simulink model "Q2_non_idealities_added"  (R2018a)
settings: Solver=FixedStepAuto  StartTime=0.0  StopTime=2  RelTol=1e-3
libraries: powerlib x14, powerlib_meascontrol x4, pePowerMeasurement x2
settings Model: Creator=ROG  LastModifiedBy=Pc

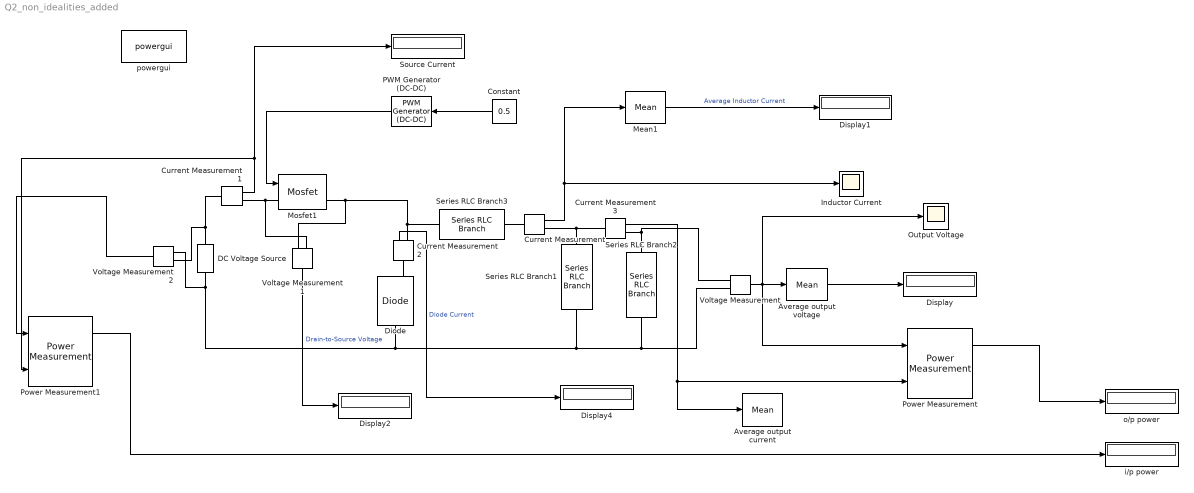
== system Q2_non_idealities_added ==
  "Average output current " : powerlib_meascontrol/Measurements/Mean  Freq=50  Vinit=0  Ts=0
  Average output voltage : powerlib_meascontrol/Measurements/Mean  Freq=50  Vinit=0  Ts=0
  Constant : Constant  Value=0.5
  Current Measurement{,1..3} (4 alike) : powerlib/Measurements/Current Measurement  PhasorSimulation=off  OutputType=Complex  PSBequivalent=0
  DC Voltage Source : powerlib/Electrical Sources/DC Voltage Source  Amplitude=56  Measurements=None
  Diode : powerlib/Power Electronics/Diode  Ron=0.001  Lon=0  Vf=0.8  IC=0  UseSnubber=0  Rs=500  Cs=250e-9  Measurements=on
  Display{,1..2,4} (4 alike) : Display
  Inductor Current : Scope
  Mean1 : powerlib_meascontrol/Measurements/Mean  Freq=50  Vinit=0  Ts=0
  Mosfet1 : powerlib/Power Electronics/Mosfet  Ron=0.022  Lon=0  Rd=0.01  Vfd=0.9  IC=0  Rs=1e5  Cs=inf  Measurements=on
  Output Voltage : Scope
  PWM Generator (DC-DC) : powerlib_meascontrol/Pulse & Signal Generators/PWM Generator (DC-DC)  Fsw=20000  Ts=0
  Power Measurement : pePowerMeasurement/Power Measurement  OverrideUsingVariant=Continuous  F=60  K=[0 1 2 3]  Ts=0
  Power Measurement1 : pePowerMeasurement/Power Measurement  OverrideUsingVariant=Continuous  F=60  K=[0 1 2 3]  Ts=0
  Series RLC Branch1 : powerlib/Elements/Series RLC Branch  LConnTagsString=__new0  RConnTagsString=__new0  BranchType=RC  Resistance=0.06  Inductance=1e-3  SetiL0=off  InitialCurrent=0  Capacitance=68e-5  Setx0=off  InitialVoltage=0  Measurements=None
  Series RLC Branch2 : powerlib/Elements/Series RLC Branch  LConnTagsString=__new0  RConnTagsString=__new0  BranchType=R  Resistance=4  Inductance=1e-3  SetiL0=off  InitialCurrent=0  Capacitance=1e-6  Setx0=off  InitialVoltage=0  Measurements=None
  Series RLC Branch3 : powerlib/Elements/Series RLC Branch  LConnTagsString=__new0  RConnTagsString=__new0  BranchType=RL  Resistance=0.064  Inductance=47e-05  SetiL0=off  InitialCurrent=0  Capacitance=1e-6  Setx0=off  InitialVoltage=0  Measurements=None
  Source Current : Display
  Voltage Measurement : powerlib/Measurements/Voltage Measurement  PhasorSimulation=off  OutputType=Complex  PSBequivalent=0
  Voltage Measurement1 : powerlib/Measurements/Voltage Measurement  PhasorSimulation=off  OutputType=Complex  PSBequivalent=0
  Voltage Measurement2 : powerlib/Measurements/Voltage Measurement  PhasorSimulation=off  OutputType=Complex  PSBequivalent=0
  i/p power : Display
  o/p power : Display
  powergui : powerlib/powergui  Priority=1  SimulationMode=Discrete  SampleTime=1e-6  frequency=60  Iterations=50  frequencyindice=0  Pbase=100e6  ErrMax=1e-4  UnitsV=kV  UnitsW=MW  buscounter=0  FunctionMessages=off  echomessages=off  EnableUseOfTLC=off  CurrentSourceSwitches=off  DisableSnubberDevices=off  DisableRonSwitches=off  DisableVfSwitches=off  DisplayEquations=off  SolverType=Tustin/Backward Euler (TBE)  Interpol=off  ExternalGateDelay=off  methode=off  Ts=100  x0status=blocks  SPID=off  SwTol=0  HookPort=off  RestoreLinks=warning  ResistiveCurrentMeasurement=off  Frange=[0:2:500]  Ylog=off  Xlog=on  ShowGrid=off  save=off  variable=ZData  structure=0  ZoomFFT=off  StartTime=0.0  cycles=1  DisplayStyle=1  fundamental=60  FreqAxis=off  MaxFrequency=1000  frequencyindicesteady=1  RmsSteady=1  display=off
  wires:
  Constant/1 -> PWM Generator (DC-DC)/1
  Voltage Measurement/1 -> Power Measurement/1, Output Voltage/1, Average output voltage/1
  Average output voltage/1 -> Display/1
  Current Measurement/1 -> Mean1/1, Inductor Current/1
  PWM Generator (DC-DC)/1 -> Mosfet1/1
  Mean1/1 -> Display1/1  "Average Inductor Current"
  Current Measurement1/1 -> Power Measurement1/2, Source Current/1
  Current Measurement2/1 -> Display4/1  "Diode Current"
  Voltage Measurement1/1 -> Display2/1  "Drain-to-Source Voltage"
  Current Measurement3/1 -> Power Measurement/2, "Average output current "/1
  Power Measurement/1 -> o/p power/1
  Voltage Measurement2/1 -> Power Measurement1/1
  Power Measurement1/1 -> i/p power/1
  connections:
  Series RLC Branch2/RConn1 -- Voltage Measurement/LConn2 -- Series RLC Branch1/RConn1 -- Diode/LConn1 -- Voltage Measurement2/LConn2 -- DC Voltage Source/LConn1
  Current Measurement/RConn1 -- Current Measurement3/LConn1 -- Series RLC Branch1/LConn1
  Mosfet1/RConn1 -- Voltage Measurement1/LConn2 -- Current Measurement2/RConn1 -- Series RLC Branch3/RConn1
  Current Measurement/LConn1 -- Series RLC Branch3/LConn1
  Mosfet1/LConn1 -- Voltage Measurement1/LConn1 -- Current Measurement1/RConn1
  Current Measurement1/LConn1 -- Voltage Measurement2/LConn1 -- DC Voltage Source/RConn1
  Current Measurement2/LConn1 -- Diode/RConn1
  Voltage Measurement/LConn1 -- Current Measurement3/RConn1 -- Series RLC Branch2/LConn1
